simulink library "halout"  (R2021b)
settings: Solver=VariableStepAuto  StartTime=0.0  StopTime=10.0  RelTol=1e-3
undefined symbols (not defined in the file): C_TASK_5MS_S, FALSE, KHAL_CAN1FD1APS3E2E_flg, KHAL_CAN1FD1APS3TxReq_flg, KHAL_CAN1FD1VCU2E2E_flg, KHAL_CAN1FD1VCU2TxReq_flg, KHAL_CAN1FD1VCU3E2E_flg, KHAL_CAN1FD1VCU3TxReq_flg, KHAL_CAN1TxReq_flg, KHAL_CAN1VMCFCM1E2E_flg, KHAL_CAN1VMCFCM1TxReq_flg, KHAL_CAN2TxReq_flg, KHAL_CAN3FD3VCU1toNIDECTxReq_flg, KHAL_CAN3FD3VCU1TxReq_flg, KHAL_CAN3FD3VCU2E2E_flg, KHAL_CAN3FD3VCU2toNIDECE2E_flg, KHAL_CAN3FD3VCU2toNIDECTxReq_flg, KHAL_CAN3FD3VCU2TxReq_flg, KHAL_CAN3TxReq_flg, KHAL_CAN4FD4CE1000E2E_flg, KHAL_CAN4FD4CE1000TxReq_flg, KHAL_CAN4TxReq_flg, KHAL_CAN5TxReq_flg, KHAL_CAN6FD6APS3E2E_flg, KHAL_CAN6FD6APS3TxReq_flg, KHAL_CAN6FD6VCU2E2E_flg, KHAL_CAN6FD6VCU2TxReq_flg, KHAL_CAN6TxReq_flg, ONE_INT, TRUE, ZERO_INT
libraries: FVT_lib x500, simulink x235
(part 13 of 25)

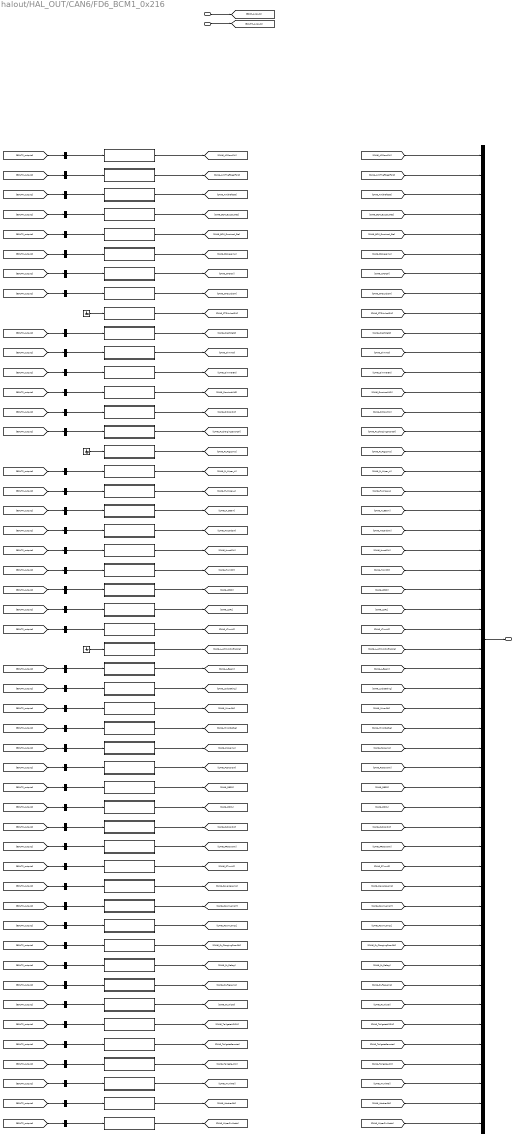
== system halout/HAL_OUT/CAN6/FD6_BCM1_0x216 ==
  BSCP_outputs : Inport  OutDataTypeStr=Bus: BSCP_outputs
  BOUTP_outputs : Inport  Port=2  OutDataTypeStr=Bus: BOUTP_outputs
  AllDoorSW : Subsystem
  AntiTheftSeatFold : Subsystem
  AntitheftSta : Subsystem
  BCMBuzzerReq : Subsystem
  BCMDoorLockSta : Subsystem
  BrakeLamp : Subsystem
  CTDCtrl : Subsystem
  CTDLockSW : Subsystem
  CTDUnlockSW : Subsystem
  CrashDetd : Subsystem
  Dimmer : Subsystem
  DimmerEN : Subsystem
  DoorLockIND : Subsystem
  DrDoorSW : Subsystem
  FrChargingDoorCtrl : Subsystem
  FrFogLamp : Subsystem
  FrWiperH : Subsystem
  FrWiperL : Subsystem
  Ground : Ground
  Ground1 : Ground
  Ground2 : Ground
  HBeam : Subsystem
  HazardSW : Subsystem
  HoodSW : Subsystem
  HornCtrl : Subsystem
  LAPMWdwEnable : Subsystem
  LBSD : Subsystem
  LBeam : Subsystem
  LDRL : Subsystem
  LTurnLP : Subsystem
  LockSetting : Subsystem
  MirrorCtrl : Subsystem
  MirrorDefog : Subsystem
  PosLamp : Subsystem
  PsDoorSW : Subsystem
  RBSD : Subsystem
  RDRL : Subsystem
  RLDoorSW : Subsystem
  RRDoorSW : Subsystem
  RTurnLP : Subsystem
  ReverseLamp : Subsystem
  RoomLampH : Subsystem
  RoomLampL : Subsystem
  RrChargingDoorCtrl : Subsystem
  RrDefog : Subsystem
  RrFogLamp : Subsystem
  RrWiper : Subsystem
  TailgateHDSW : Subsystem
  TailgateRemote : Subsystem
  TailgateSW : Subsystem
  TrunkRel : Subsystem
  WasherCtrl : Subsystem
  WiperFixMode : Subsystem
  bus_creator : BusCreator  Inputs=50  OutDataTypeStr=Bus: DT_CAN6_SG_FD6_BCM1  NonVirtualBus=on
  bus_selector : BusSelector  OutputSignals=VOUTP_AllDoorSW_flg
  bus_selector1 : BusSelector  OutputSignals=VOUTP_AntitheftSeatFlod_flg
  bus_selector10 : BusSelector  OutputSignals=VOUTP_DimmerEN_flg
  bus_selector11 : BusSelector  OutputSignals=VOUTP_DoorLockIND_flg
  bus_selector12 : BusSelector  OutputSignals=VOUTP_DrDoorSW_flg
  bus_selector13 : BusSelector  OutputSignals=VOUTP_FrChargingDoorCtrl_enum
  bus_selector14 : BusSelector  OutputSignals=VOUTP_FrWiperH_flg
  bus_selector15 : BusSelector  OutputSignals=VOUTP_FrWiperL_flg
  bus_selector16 : BusSelector  OutputSignals=VOUTP_HBeam_flg
  bus_selector17 : BusSelector  OutputSignals=VOUTP_HazardSW_flg
  bus_selector18 : BusSelector  OutputSignals=VOUTP_HoodSW_flg
  bus_selector19 : BusSelector  OutputSignals=VOUTP_HornCtrl_flg
  bus_selector2 : BusSelector  OutputSignals=VOUTP_AntitheftSta_enum
  bus_selector20 : BusSelector  OutputSignals=VOUTP_LBSD_flg
  bus_selector21 : BusSelector  OutputSignals=VOUTP_LDRL_flg
  bus_selector22 : BusSelector  OutputSignals=VOUTP_LTurnLP_flg
  bus_selector23 : BusSelector  OutputSignals=VOUTP_LBeam_flg
  bus_selector24 : BusSelector  OutputSignals=VOUTP_LockSetting_flg
  bus_selector25 : BusSelector  OutputSignals=VOUTP_MirrorCtrl_enum
  bus_selector26 : BusSelector  OutputSignals=VOUTP_MirrorDefog_flg
  bus_selector27 : BusSelector  OutputSignals=VOUTP_PosLamp_flg
  bus_selector28 : BusSelector  OutputSignals=VOUTP_PsDoorSW_flg
  bus_selector29 : BusSelector  OutputSignals=VOUTP_RBSD_flg
  bus_selector3 : BusSelector  OutputSignals=VOUTP_BCMBuzzerReq_flg
  bus_selector30 : BusSelector  OutputSignals=VOUTP_RDRL_flg
  bus_selector31 : BusSelector  OutputSignals=VOUTP_RLDoorSW_flg
  bus_selector32 : BusSelector  OutputSignals=VOUTP_RRDoorSW_flg
  bus_selector33 : BusSelector  OutputSignals=VOUTP_RTurnLP_flg
  bus_selector34 : BusSelector  OutputSignals=VOUTP_ReverseLamp_flg
  bus_selector35 : BusSelector  OutputSignals=VOUTP_RoomLampH_flg
  bus_selector36 : BusSelector  OutputSignals=VOUTP_RoomLampL_flg
  bus_selector37 : BusSelector  OutputSignals=VOUTP_RrChargingDoorCtrl_enum
  bus_selector38 : BusSelector  OutputSignals=VOUTP_RrDefog_flg
  bus_selector39 : BusSelector  OutputSignals=VOUTP_RrFogLamp_flg
  bus_selector4 : BusSelector  OutputSignals=VOUTP_BCMDoorLockSta_flg
  bus_selector40 : BusSelector  OutputSignals=VOUTP_RrWiper_flg
  bus_selector41 : BusSelector  OutputSignals=VOUTP_TailgateHDSW_flg
  bus_selector42 : BusSelector  OutputSignals=VOUTP_TailgateRemote_enum
  bus_selector43 : BusSelector  OutputSignals=VOUTP_TailgateSW_flg
  bus_selector44 : BusSelector  OutputSignals=VOUTP_TrunkRel_flg
  bus_selector45 : BusSelector  OutputSignals=VOUTP_WasherCtrl_enum
  bus_selector46 : BusSelector  OutputSignals=VOUTP_WiperFixMode_flg
  bus_selector5 : BusSelector  OutputSignals=VOUTP_BrakeLamp_flg
  bus_selector6 : BusSelector  OutputSignals=VOUTP_CTDCtrl_enum
  bus_selector7 : BusSelector  OutputSignals=VOUTP_CTDLockSW_flg
  bus_selector8 : BusSelector  OutputSignals=VOUTP_CrashDetd_flg
  bus_selector9 : BusSelector  OutputSignals=VOUTP_Dimmer_pct
  FD6_BCM1 : Outport
  wires:
  BSCP_outputs/1 -> [BSCP_outputs]
  BOUTP_outputs/1 -> [BOUTP_outputs]
  [CAN6_AllDoorSW] -> bus_creator/1  "CAN6_AllDoorSW"
  [CAN6_AntiTheftSeatFold] -> bus_creator/2  "CAN6_AntiTheftSeatFold"
  [CAN6_AntitheftSta] -> bus_creator/3  "CAN6_AntitheftSta"
  [CAN6_BCM_Buzzer_Req] -> bus_creator/4  "CAN6_BCM_Buzzer_Req"
  [CAN6_BCM_DoorLock_Sta] -> bus_creator/5  "CAN6_BCM_DoorLock_Sta"
  [CAN6_BrakeLamp] -> bus_creator/6  "CAN6_BrakeLamp"
  [CAN6_CTDCtrl] -> bus_creator/7  "CAN6_CTDCtrl"
  [CAN6_CTDLockSW] -> bus_creator/8  "CAN6_CTDLockSW"
  [CAN6_CTDUnlockSW] -> bus_creator/9  "CAN6_CTDUnlockSW"
  [CAN6_CrashDetd] -> bus_creator/10  "CAN6_CrashDetd"
  [CAN6_Dimmer] -> bus_creator/11  "CAN6_Dimmer"
  [CAN6_DimmerEN] -> bus_creator/12  "CAN6_DimmerEN"
  [CAN6_DoorLockIND] -> bus_creator/13  "CAN6_DoorLockIND"
  [CAN6_DrDoorSW] -> bus_creator/14  "CAN6_DrDoorSW"
  [CAN6_Fr_ChargingDoorCtrl] -> bus_creator/15  "CAN6_Fr_ChargingDoorCtrl"
  [CAN6_Fr_FogLamp] -> bus_creator/16  "CAN6_Fr_FogLamp"
  [CAN6_Fr_Wiper_H] -> bus_creator/17  "CAN6_Fr_Wiper_H"
  [CAN6_Fr_Wiper_L] -> bus_creator/18  "CAN6_Fr_Wiper_L"
  [CAN6_H_Beam] -> bus_creator/19  "CAN6_H_Beam"
  [CAN6_HazardSW] -> bus_creator/20  "CAN6_HazardSW"
  [CAN6_HoodSW] -> bus_creator/21  "CAN6_HoodSW"
  [CAN6_HornCtrl] -> bus_creator/22  "CAN6_HornCtrl"
  [CAN6_LBSD] -> bus_creator/23  "CAN6_LBSD"
  [CAN6_LDRL] -> bus_creator/24  "CAN6_LDRL"
  [CAN6_LTurnLP] -> bus_creator/25  "CAN6_LTurnLP"
  [CAN6_L_APM_WdwEnable] -> bus_creator/26  "CAN6_L_APM_WdwEnable"
  [CAN6_L_Beam] -> bus_creator/27  "CAN6_L_Beam"
  [CAN6_LockSetting] -> bus_creator/28  "CAN6_LockSetting"
  [CAN6_MirrorCtrl] -> bus_creator/29  "CAN6_MirrorCtrl"
  [CAN6_MirrorDefog] -> bus_creator/30  "CAN6_MirrorDefog"
  [CAN6_PosLamp] -> bus_creator/31  "CAN6_PosLamp"
  [CAN6_PsDoorSW] -> bus_creator/32  "CAN6_PsDoorSW"
  [CAN6_RBSD] -> bus_creator/33  "CAN6_RBSD"
  [CAN6_RDRL] -> bus_creator/34  "CAN6_RDRL"
  [CAN6_RLDoorSW] -> bus_creator/35  "CAN6_RLDoorSW"
  [CAN6_RRDoorSW] -> bus_creator/36  "CAN6_RRDoorSW"
  [CAN6_RTurnLP] -> bus_creator/37  "CAN6_RTurnLP"
  [CAN6_ReverseLamp] -> bus_creator/38  "CAN6_ReverseLamp"
  [CAN6_RoomLampH] -> bus_creator/39  "CAN6_RoomLampH"
  [CAN6_RoomLampL] -> bus_creator/40  "CAN6_RoomLampL"
  [CAN6_Rr_ChargingDoorCtrl] -> bus_creator/41  "CAN6_Rr_ChargingDoorCtrl"
  [CAN6_Rr_Defog] -> bus_creator/42  "CAN6_Rr_Defog"
  [CAN6_Rr_FogLamp] -> bus_creator/43  "CAN6_Rr_FogLamp"
  [CAN6_Rr_Wiper] -> bus_creator/44  "CAN6_Rr_Wiper"
  [CAN6_TailgateHDSW] -> bus_creator/45  "CAN6_TailgateHDSW"
  [CAN6_TailgateRemote] -> bus_creator/46  "CAN6_TailgateRemote"
  [CAN6_Tailgate_SW] -> bus_creator/47  "CAN6_Tailgate_SW"
  [CAN6_TrunkRel] -> bus_creator/48  "CAN6_TrunkRel"
  [CAN6_WasherCtrl] -> bus_creator/49  "CAN6_WasherCtrl"
  [CAN6_WiperFixMode] -> bus_creator/50  "CAN6_WiperFixMode"
  bus_creator/1 -> FD6_BCM1/1
  AllDoorSW/1(CAN6_AllDoorSW) -> [CAN6_AllDoorSW]
  AntiTheftSeatFold/1(CAN6_AntiTheftSeatFold) -> [CAN6_AntiTheftSeatFold]
  AntitheftSta/1(CAN6_AntitheftSta) -> [CAN6_AntitheftSta]
  BCMBuzzerReq/1(CAN6_BCM_Buzzer_Req) -> [CAN6_BCM_Buzzer_Req]
  BCMDoorLockSta/1(CAN6_BCM_DoorLock_Sta) -> [CAN6_BCM_DoorLock_Sta]
  BrakeLamp/1(CAN6_BrakeLamp) -> [CAN6_BrakeLamp]
  CTDCtrl/1(CAN6_CTDCtrl) -> [CAN6_CTDCtrl]
  CTDLockSW/1(CAN6_CTDLockSW) -> [CAN6_CTDLockSW]
  CTDUnlockSW/1(CAN6_CTDUnlockSW) -> [CAN6_CTDUnlockSW]
  CrashDetd/1(CAN6_CrashDetd) -> [CAN6_CrashDetd]
  Dimmer/1(CAN6_Dimmer) -> [CAN6_Dimmer]
  DimmerEN/1(CAN6_DimmerEN) -> [CAN6_DimmerEN]
  DoorLockIND/1(CAN6_DoorLockIND) -> [CAN6_DoorLockIND]
  DrDoorSW/1(CAN6_DrDoorSW) -> [CAN6_DrDoorSW]
  FrChargingDoorCtrl/1(CAN6_Fr_ChargingDoorCtrl) -> [CAN6_Fr_ChargingDoorCtrl]
  FrFogLamp/1(CAN6_Fr_FogLamp) -> [CAN6_Fr_FogLamp]
  FrWiperH/1(CAN6_Fr_Wiper_H) -> [CAN6_Fr_Wiper_H]
  FrWiperL/1(CAN6_Fr_Wiper_L) -> [CAN6_Fr_Wiper_L]
  HBeam/1(CAN6_H_Beam) -> [CAN6_H_Beam]
  HazardSW/1(CAN6_HazardSW) -> [CAN6_HazardSW]
  HoodSW/1(CAN6_HoodSW) -> [CAN6_HoodSW]
  HornCtrl/1(CAN6_HornCtrl) -> [CAN6_HornCtrl]
  LBSD/1(CAN6_LBSD) -> [CAN6_LBSD]
  LDRL/1(CAN6_LDRL) -> [CAN6_LDRL]
  LTurnLP/1(CAN6_LTurnLP) -> [CAN6_LTurnLP]
  LAPMWdwEnable/1(CAN6_L_APM_WdwEnable) -> [CAN6_L_APM_WdwEnable]
  LBeam/1(CAN6_L_Beam) -> [CAN6_L_Beam]
  LockSetting/1(CAN6_LockSetting) -> [CAN6_LockSetting]
  MirrorCtrl/1(CAN6_MirrorCtrl) -> [CAN6_MirrorCtrl]
  MirrorDefog/1(CAN6_MirrorDefog) -> [CAN6_MirrorDefog]
  PosLamp/1(CAN6_PosLamp) -> [CAN6_PosLamp]
  PsDoorSW/1(CAN6_PsDoorSW) -> [CAN6_PsDoorSW]
  RBSD/1(CAN6_RBSD) -> [CAN6_RBSD]
  RDRL/1(CAN6_RDRL) -> [CAN6_RDRL]
  RLDoorSW/1(CAN6_RLDoorSW) -> [CAN6_RLDoorSW]
  RRDoorSW/1(CAN6_RRDoorSW) -> [CAN6_RRDoorSW]
  RTurnLP/1(CAN6_RTurnLP) -> [CAN6_RTurnLP]
  ReverseLamp/1(CAN6_ReverseLamp) -> [CAN6_ReverseLamp]
  RoomLampH/1(CAN6_RoomLampH) -> [CAN6_RoomLampH]
  RoomLampL/1(CAN6_RoomLampL) -> [CAN6_RoomLampL]
  RrChargingDoorCtrl/1(CAN6_Rr_ChargingDoorCtrl) -> [CAN6_Rr_ChargingDoorCtrl]
  RrDefog/1(CAN6_Rr_Defog) -> [CAN6_Rr_Defog]
  RrFogLamp/1(CAN6_Rr_FogLamp) -> [CAN6_Rr_FogLamp]
  RrWiper/1(CAN6_Rr_Wiper) -> [CAN6_Rr_Wiper]
  TailgateHDSW/1(CAN6_TailgateHDSW) -> [CAN6_TailgateHDSW]
  TailgateRemote/1(CAN6_TailgateRemote) -> [CAN6_TailgateRemote]
  TailgateSW/1(CAN6_Tailgate_SW) -> [CAN6_Tailgate_SW]
  TrunkRel/1(CAN6_TrunkRel) -> [CAN6_TrunkRel]
  WasherCtrl/1(CAN6_WasherCtrl) -> [CAN6_WasherCtrl]
  WiperFixMode/1(CAN6_WiperFixMode) -> [CAN6_WiperFixMode]
  bus_selector/1 -> AllDoorSW/1(AllDoorSW)  "<VOUTP_AllDoorSW_flg>"
  [BOUTP_outputs] -> bus_selector/1
  bus_selector1/1 -> AntiTheftSeatFold/1(AntiTheftSeatFold)  "<VOUTP_AntitheftSeatFlod_flg>"
  [BOUTP_outputs] -> bus_selector1/1
  bus_selector2/1 -> AntitheftSta/1(AntitheftSta)  "<VOUTP_AntitheftSta_enum>"
  [BOUTP_outputs] -> bus_selector2/1
  bus_selector3/1 -> BCMBuzzerReq/1(BCMBuzzerReq)  "<VOUTP_BCMBuzzerReq_flg>"
  [BOUTP_outputs] -> bus_selector3/1
  bus_selector4/1 -> BCMDoorLockSta/1(BCMDoorLockSta)  "<VOUTP_BCMDoorLockSta_flg>"
  [BOUTP_outputs] -> bus_selector4/1
  bus_selector5/1 -> BrakeLamp/1(BrakeLamp)  "<VOUTP_BrakeLamp_flg>"
  [BOUTP_outputs] -> bus_selector5/1
  bus_selector6/1 -> CTDCtrl/1(CTDCtrl)  "<VOUTP_CTDCtrl_enum>"
  [BOUTP_outputs] -> bus_selector6/1
  bus_selector7/1 -> CTDLockSW/1(CTDLockSW)  "<VOUTP_CTDLockSW_flg>"
  [BOUTP_outputs] -> bus_selector7/1
  Ground/1 -> CTDUnlockSW/1(CTDUnlockSW)
  bus_selector8/1 -> CrashDetd/1(CrashDetd)  "<VOUTP_CrashDetd_flg>"
  [BOUTP_outputs] -> bus_selector8/1
  bus_selector9/1 -> Dimmer/1(Dimmer)  "<VOUTP_Dimmer_pct>"
  [BOUTP_outputs] -> bus_selector9/1
  bus_selector10/1 -> DimmerEN/1(DimmerEN)  "<VOUTP_DimmerEN_flg>"
  [BOUTP_outputs] -> bus_selector10/1
  bus_selector11/1 -> DoorLockIND/1(DoorLockIND)  "<VOUTP_DoorLockIND_flg>"
  [BOUTP_outputs] -> bus_selector11/1
  bus_selector12/1 -> DrDoorSW/1(DrDoorSW)  "<VOUTP_DrDoorSW_flg>"
  [BOUTP_outputs] -> bus_selector12/1
  bus_selector13/1 -> FrChargingDoorCtrl/1(FrChargingDoorCtrl)  "<VOUTP_FrChargingDoorCtrl_enum>"
  [BOUTP_outputs] -> bus_selector13/1
  Ground1/1 -> FrFogLamp/1(FrFogLamp)
  bus_selector14/1 -> FrWiperH/1(FrWiperH)  "<VOUTP_FrWiperH_flg>"
  [BOUTP_outputs] -> bus_selector14/1
  bus_selector15/1 -> FrWiperL/1(FrWiperL)  "<VOUTP_FrWiperL_flg>"
  [BOUTP_outputs] -> bus_selector15/1
  bus_selector16/1 -> HBeam/1(HBeam)  "<VOUTP_HBeam_flg>"
  [BOUTP_outputs] -> bus_selector16/1
  bus_selector17/1 -> HazardSW/1(HazardSW)  "<VOUTP_HazardSW_flg>"
  [BOUTP_outputs] -> bus_selector17/1
  bus_selector18/1 -> HoodSW/1(HoodSW)  "<VOUTP_HoodSW_flg>"
  [BOUTP_outputs] -> bus_selector18/1
  bus_selector19/1 -> HornCtrl/1(HornCtrl)  "<VOUTP_HornCtrl_flg>"
  [BOUTP_outputs] -> bus_selector19/1
  bus_selector20/1 -> LBSD/1(LBSD)  "<VOUTP_LBSD_flg>"
  [BOUTP_outputs] -> bus_selector20/1
  bus_selector21/1 -> LDRL/1(LDRL)  "<VOUTP_LDRL_flg>"
  [BOUTP_outputs] -> bus_selector21/1
  bus_selector22/1 -> LTurnLP/1(LTurnLP)  "<VOUTP_LTurnLP_flg>"
  [BOUTP_outputs] -> bus_selector22/1
  Ground2/1 -> LAPMWdwEnable/1(LAPMWdwEnable)
  bus_selector23/1 -> LBeam/1(LBeam)  "<VOUTP_LBeam_flg>"
  [BOUTP_outputs] -> bus_selector23/1
  bus_selector24/1 -> LockSetting/1(LockSetting)  "<VOUTP_LockSetting_flg>"
  [BOUTP_outputs] -> bus_selector24/1
  bus_selector25/1 -> MirrorCtrl/1(MirrorCtrl)  "<VOUTP_MirrorCtrl_enum>"
  [BOUTP_outputs] -> bus_selector25/1
  bus_selector26/1 -> MirrorDefog/1(MirrorDefog)  "<VOUTP_MirrorDefog_flg>"
  [BOUTP_outputs] -> bus_selector26/1
  bus_selector27/1 -> PosLamp/1(PosLamp)  "<VOUTP_PosLamp_flg>"
  [BOUTP_outputs] -> bus_selector27/1
  bus_selector28/1 -> PsDoorSW/1(PsDoorSW)  "<VOUTP_PsDoorSW_flg>"
  [BOUTP_outputs] -> bus_selector28/1
  bus_selector29/1 -> RBSD/1(RBSD)  "<VOUTP_RBSD_flg>"
  [BOUTP_outputs] -> bus_selector29/1
  bus_selector30/1 -> RDRL/1(RDRL)  "<VOUTP_RDRL_flg>"
  [BOUTP_outputs] -> bus_selector30/1
  bus_selector31/1 -> RLDoorSW/1(RLDoorSW)  "<VOUTP_RLDoorSW_flg>"
  [BOUTP_outputs] -> bus_selector31/1
  bus_selector32/1 -> RRDoorSW/1(RRDoorSW)  "<VOUTP_RRDoorSW_flg>"
  [BOUTP_outputs] -> bus_selector32/1
  bus_selector33/1 -> RTurnLP/1(RTurnLP)  "<VOUTP_RTurnLP_flg>"
  [BOUTP_outputs] -> bus_selector33/1
  bus_selector34/1 -> ReverseLamp/1(ReverseLamp)  "<VOUTP_ReverseLamp_flg>"
  [BOUTP_outputs] -> bus_selector34/1
  bus_selector35/1 -> RoomLampH/1(RoomLampH)  "<VOUTP_RoomLampH_flg>"
  [BOUTP_outputs] -> bus_selector35/1
  bus_selector36/1 -> RoomLampL/1(RoomLampL)  "<VOUTP_RoomLampL_flg>"
  [BOUTP_outputs] -> bus_selector36/1
  bus_selector37/1 -> RrChargingDoorCtrl/1(RrChargingDoorCtrl)  "<VOUTP_RrChargingDoorCtrl_enum>"
  [BOUTP_outputs] -> bus_selector37/1
  bus_selector38/1 -> RrDefog/1(RrDefog)  "<VOUTP_RrDefog_flg>"
  [BOUTP_outputs] -> bus_selector38/1
  bus_selector39/1 -> RrFogLamp/1(RrFogLamp)  "<VOUTP_RrFogLamp_flg>"
  [BOUTP_outputs] -> bus_selector39/1
  bus_selector40/1 -> RrWiper/1(RrWiper)  "<VOUTP_RrWiper_flg>"
  [BOUTP_outputs] -> bus_selector40/1
  bus_selector41/1 -> TailgateHDSW/1(TailgateHDSW)  "<VOUTP_TailgateHDSW_flg>"
  [BOUTP_outputs] -> bus_selector41/1
  bus_selector42/1 -> TailgateRemote/1(TailgateRemote)  "<VOUTP_TailgateRemote_enum>"
  [BOUTP_outputs] -> bus_selector42/1
  bus_selector43/1 -> TailgateSW/1(TailgateSW)  "<VOUTP_TailgateSW_flg>"
  [BOUTP_outputs] -> bus_selector43/1
  bus_selector44/1 -> TrunkRel/1(TrunkRel)  "<VOUTP_TrunkRel_flg>"
  [BOUTP_outputs] -> bus_selector44/1
  bus_selector45/1 -> WasherCtrl/1(WasherCtrl)  "<VOUTP_WasherCtrl_enum>"
  [BOUTP_outputs] -> bus_selector45/1
  bus_selector46/1 -> WiperFixMode/1(WiperFixMode)  "<VOUTP_WiperFixMode_flg>"
  [BOUTP_outputs] -> bus_selector46/1

== system halout/HAL_OUT/CAN6/FD6_VCU1_0x116 ==
  BSCP_outputs : Inport  OutDataTypeStr=Bus: BSCP_outputs
  BOUTP_outputs : Inport  Port=2  OutDataTypeStr=Bus: BOUTP_outputs
  CCCrlSta : Subsystem
  EngAGSCloseSta : Subsystem
  EngActvDmpDisabSta : Subsystem
  EngCoastDwSta : Subsystem
  EngPwrLockSta : Subsystem
  Ground{,1..4} (5 alike) : Ground
  HVPwrSta : Subsystem
  LVPwrSta : Subsystem
  MSACrlSta : Subsystem
  PButtonSta : Subsystem
  PrkReq : Subsystem
  PrkReqValid : Subsystem
  PwrSta : Subsystem
  ShiftGearPosn : Subsystem
  VehMalfunLevel : Subsystem
  XWDMode : Subsystem
  bus_creator : BusCreator  Inputs=15  OutDataTypeStr=Bus: DT_CAN6_SG_FD6_VCU1  NonVirtualBus=on
  bus_selector : BusSelector  OutputSignals=VOUTP_CCCtrlSta_enum
  bus_selector1 : BusSelector  OutputSignals=VOUTP_IVIPwrLockSta_enum
  bus_selector2 : BusSelector  OutputSignals=VOUTP_HVPwrSta_flg
  bus_selector3 : BusSelector  OutputSignals=VOUTP_LVPwrSta_flg
  bus_selector4 : BusSelector  OutputSignals=VOUTP_MSACtrlSta_enum
  bus_selector5 : BusSelector  OutputSignals=VOUTP_PButtonSta_enum
  bus_selector6 : BusSelector  OutputSignals=VOUTP_ActParkRequest_flg
  bus_selector7 : BusSelector  OutputSignals=VOUTP_PowerSta_enum
  bus_selector8 : BusSelector  OutputSignals=VOUTP_ShiftGearPosn_enum
  bus_selector9 : BusSelector  OutputSignals=VOUTP_DrivetrainSelect_enum
  FD6_VCU1 : Outport
  wires:
  BSCP_outputs/1 -> [BSCP_outputs]
  BOUTP_outputs/1 -> [BOUTP_outputs]
  [CAN6_CC_Crl_Sta] -> bus_creator/1  "CAN6_CC_Crl_Sta"
  [CAN6_Eng_AGSCloseSta] -> bus_creator/2  "CAN6_Eng_AGSCloseSta"
  [CAN6_Eng_ActvDmpDisabSta] -> bus_creator/3  "CAN6_Eng_ActvDmpDisabSta"
  [CAN6_Eng_CoastDwSta] -> bus_creator/4  "CAN6_Eng_CoastDwSta"
  [CAN6_Eng_PwrLockSta] -> bus_creator/5  "CAN6_Eng_PwrLockSta"
  [CAN6_HVPwrSta] -> bus_creator/6  "CAN6_HVPwrSta"
  [CAN6_LVPwrSta] -> bus_creator/7  "CAN6_LVPwrSta"
  [CAN6_MSA_Crl_Sta] -> bus_creator/8  "CAN6_MSA_Crl_Sta"
  [CAN6_P_Button_Sta] -> bus_creator/9  "CAN6_P_Button_Sta"
  [CAN6_PrkReq] -> bus_creator/10  "CAN6_PrkReq"
  [CAN6_PrkReqValid] -> bus_creator/11  "CAN6_PrkReqValid"
  [CAN6_PwrSta] -> bus_creator/12  "CAN6_PwrSta"
  [CAN6_ShiftGearPosn] -> bus_creator/13  "CAN6_ShiftGearPosn"
  [CAN6_VehMalfunLevel] -> bus_creator/14  "CAN6_VehMalfunLevel"
  [CAN6_XWDMode] -> bus_creator/15  "CAN6_XWDMode"
  bus_creator/1 -> FD6_VCU1/1
  CCCrlSta/1(CAN6_CC_Crl_Sta) -> [CAN6_CC_Crl_Sta]
  EngAGSCloseSta/1(CAN6_Eng_AGSCloseSta) -> [CAN6_Eng_AGSCloseSta]
  EngActvDmpDisabSta/1(CAN6_Eng_ActvDmpDisabSta) -> [CAN6_Eng_ActvDmpDisabSta]
  EngCoastDwSta/1(CAN6_Eng_CoastDwSta) -> [CAN6_Eng_CoastDwSta]
  EngPwrLockSta/1(CAN6_Eng_PwrLockSta) -> [CAN6_Eng_PwrLockSta]
  HVPwrSta/1(CAN6_HVPwrSta) -> [CAN6_HVPwrSta]
  LVPwrSta/1(CAN6_LVPwrSta) -> [CAN6_LVPwrSta]
  MSACrlSta/1(CAN6_MSA_Crl_Sta) -> [CAN6_MSA_Crl_Sta]
  PButtonSta/1(CAN6_P_Button_Sta) -> [CAN6_P_Button_Sta]
  PrkReq/1(CAN6_PrkReq) -> [CAN6_PrkReq]
  PrkReqValid/1(CAN6_PrkReqValid) -> [CAN6_PrkReqValid]
  PwrSta/1(CAN6_PwrSta) -> [CAN6_PwrSta]
  ShiftGearPosn/1(CAN6_ShiftGearPosn) -> [CAN6_ShiftGearPosn]
  VehMalfunLevel/1(CAN6_VehMalfunLevel) -> [CAN6_VehMalfunLevel]
  XWDMode/1(CAN6_XWDMode) -> [CAN6_XWDMode]
  bus_selector/1 -> CCCrlSta/1(CCCrlSta)  "<VOUTP_CCCtrlSta_enum>"
  [BOUTP_outputs] -> bus_selector/1
  Ground/1 -> EngAGSCloseSta/1(EngAGSCloseSta)
  Ground1/1 -> EngActvDmpDisabSta/1(EngActvDmpDisabSta)
  Ground2/1 -> EngCoastDwSta/1(EngCoastDwSta)
  bus_selector1/1 -> EngPwrLockSta/1(EngPwrLockSta)  "<VOUTP_IVIPwrLockSta_enum>"
  [BOUTP_outputs] -> bus_selector1/1
  bus_selector2/1 -> HVPwrSta/1(HVPwrSta)  "<VOUTP_HVPwrSta_flg>"
  [BOUTP_outputs] -> bus_selector2/1
  bus_selector3/1 -> LVPwrSta/1(LVPwrSta)  "<VOUTP_LVPwrSta_flg>"
  [BOUTP_outputs] -> bus_selector3/1
  bus_selector4/1 -> MSACrlSta/1(MSACrlSta)  "<VOUTP_MSACtrlSta_enum>"
  [BOUTP_outputs] -> bus_selector4/1
  bus_selector5/1 -> PButtonSta/1(PButtonSta)  "<VOUTP_PButtonSta_enum>"
  [BOUTP_outputs] -> bus_selector5/1
  bus_selector6/1 -> PrkReq/1(PrkReq)  "<VOUTP_ActParkRequest_flg>"
  [BOUTP_outputs] -> bus_selector6/1
  Ground3/1 -> PrkReqValid/1(PrkReqValid)
  bus_selector7/1 -> PwrSta/1(PwrSta)  "<VOUTP_PowerSta_enum>"
  [BOUTP_outputs] -> bus_selector7/1
  bus_selector8/1 -> ShiftGearPosn/1(ShiftGearPosn)  "<VOUTP_ShiftGearPosn_enum>"
  [BOUTP_outputs] -> bus_selector8/1
  Ground4/1 -> VehMalfunLevel/1(VehMalfunLevel)
  bus_selector9/1 -> XWDMode/1(XWDMode)  "<VOUTP_DrivetrainSelect_enum>"
  [BOUTP_outputs] -> bus_selector9/1

== system halout/HAL_OUT/CAN6/FD6_VCU2_0x154 ==
  BSCP_outputs : Inport  OutDataTypeStr=Bus: BSCP_outputs
  BOUTP_outputs : Inport  Port=2  OutDataTypeStr=Bus: BOUTP_outputs
  Trigger : TriggerPort  TriggerType=function-call  VariantControl=(inherit)
  ACCCtrlAvail : Subsystem
  AccPedalOverride : Subsystem
  ActAPSPosn : Subsystem
  Byte_0 : Subsystem
  Byte_1 : Subsystem
  Byte_10 : Subsystem
  Byte_11 : Subsystem
  Byte_12 : Subsystem
  Byte_13 : Subsystem
  Byte_14 : Subsystem
  Byte_15 : Subsystem
  Byte_2 : Subsystem
  Byte_3 : Subsystem
  Byte_4 : Subsystem
  Byte_5 : Subsystem
  Byte_6 : Subsystem
  Byte_7 : Constant  Value=ZERO_INT
  Byte_8 : Constant  Value=ZERO_INT
  Byte_9 : Constant  Value=ZERO_INT
  CRC8_IfAction_Tx : Subsystem  AncestorBlock=FVT_lib/hal/CRC8_IfAction_Tx
      mask help: MeasumentTrigerEvent
      mask Display: fprintf('CRC8_IfAction');
  CSVCU2CAN6 : Subsystem
  Constant : Constant  Value=KHAL_CAN6FD6VCU2E2E_flg
  Constant1 : Constant  Value=0x32
  Constant2 : Constant  Value=0xBF
  Constant3 : Constant  Value=KHAL_CAN6FD6VCU2E2E_flg
  Constant4 : Constant  Value=KHAL_CAN6FD6VCU2E2E_flg
  DriverTq : Subsystem
  FrDriverTq : Subsystem
  Ground{,1..7} (8 alike) : Ground
  Mux2 : Mux  Inputs=15
  RCVCU2CAN6 : Subsystem
  RollingCounter_IfAction : FVT_lib/hal/RollingCounter_IfAction
  RollingCounter_IfAction1 : FVT_lib/hal/RollingCounter_IfAction
  RrDriverTq : Subsystem
  Terminator : Terminator
  VehActPwr : Subsystem
  bus_creator : BusCreator  Inputs=9  OutDataTypeStr=Bus: DT_CAN6_SG_FD6_VCU2  NonVirtualBus=on
  bus_selector : BusSelector  OutputSignals=VOUTP_DriverWhlTqDemFr_Nm
  bus_selector1 : BusSelector  OutputSignals=VOUTP_DriverWhlTqDemFr_Nm
  bus_selector10 : BusSelector  OutputSignals=VOUTP_DriverWhlTqDemFr_Nm
  bus_selector11 : BusSelector  OutputSignals=VOUTP_DriverWhlTqDemRr_Nm
  bus_selector2 : BusSelector  OutputSignals=VOUTP_DriverWhlTqDemRr_Nm
  bus_selector3 : BusSelector  OutputSignals=VOUTP_DriverWhlTqDemRr_Nm
  bus_selector4 : BusSelector  OutputSignals=VOUTP_ACCCtrlAvail_flg
  bus_selector5 : BusSelector  OutputSignals=VOUTP_ACCPedalOvrd_flg
  bus_selector6 : BusSelector  OutputSignals=VOUTP_ActAPSPosn_pct
  bus_selector7 : BusSelector  OutputSignals=VOUTP_ACCCtrlAvail_flg
  bus_selector8 : BusSelector  OutputSignals=VOUTP_ACCPedalOvrd_flg
  bus_selector9 : BusSelector  OutputSignals=VOUTP_ActAPSPosn_pct
  FD6_VCU2 : Outport
  wires:
  BSCP_outputs/1 -> [BSCP_outputs]
  BOUTP_outputs/1 -> [BOUTP_outputs]
  [CAN6_ACC_CtrlAvail] -> bus_creator/1  "CAN6_ACC_CtrlAvail"
  [CAN6_AccPedal_Override] -> bus_creator/2  "CAN6_AccPedal_Override"
  [CAN6_ActAPSPosn] -> bus_creator/3  "CAN6_ActAPSPosn"
  [CAN6_CS_VCU2_CAN6] -> bus_creator/4  "CAN6_CS_VCU2_CAN6"
  [CAN6_DriverTq] -> bus_creator/5  "CAN6_DriverTq"
  [CAN6_Fr_DriverTq] -> bus_creator/6  "CAN6_Fr_DriverTq"
  [CAN6_RC_VCU2_CAN6] -> bus_creator/7  "CAN6_RC_VCU2_CAN6"
  [CAN6_Rr_DriverTq] -> bus_creator/8  "CAN6_Rr_DriverTq"
  [CAN6_VehActPwr] -> bus_creator/9  "CAN6_VehActPwr"
  bus_creator/1 -> FD6_VCU2/1
  ACCCtrlAvail/1(CAN6_ACC_CtrlAvail) -> [CAN6_ACC_CtrlAvail]
  AccPedalOverride/1(CAN6_AccPedal_Override) -> [CAN6_AccPedal_Override]
  ActAPSPosn/1(CAN6_ActAPSPosn) -> [CAN6_ActAPSPosn]
  CSVCU2CAN6/1(CAN6_CS_VCU2_CAN6) -> [CAN6_CS_VCU2_CAN6]
  DriverTq/1(CAN6_DriverTq) -> [CAN6_DriverTq]
  FrDriverTq/1(CAN6_Fr_DriverTq) -> [CAN6_Fr_DriverTq]
  RCVCU2CAN6/1(CAN6_RC_VCU2_CAN6) -> [CAN6_RC_VCU2_CAN6]
  RrDriverTq/1(CAN6_Rr_DriverTq) -> [CAN6_Rr_DriverTq]
  VehActPwr/1(CAN6_VehActPwr) -> [CAN6_VehActPwr]
  Byte_0/1(Byte_0) -> Terminator/1
  Byte_1/1(Byte_1) -> [Byte_1]
  Byte_2/1(Byte_2) -> [Byte_2]
  Byte_3/1(Byte_3) -> [Byte_3]
  Byte_4/1(Byte_4) -> [Byte_4]
  Byte_5/1(Byte_5) -> [Byte_5]
  Byte_6/1(Byte_6) -> [Byte_6]
  Byte_7/1 -> [Byte_7]
  Byte_8/1 -> [Byte_8]
  Byte_9/1 -> [Byte_9]
  Byte_10/1(Byte_10) -> [Byte_10]
  Byte_11/1(Byte_11) -> [Byte_11]
  Byte_12/1(Byte_12) -> [Byte_12]
  Byte_13/1(Byte_13) -> [Byte_13]
  Byte_14/1(Byte_14) -> [Byte_14]
  Byte_15/1(Byte_15) -> [Byte_15]
  Mux2/1 -> CRC8_IfAction_Tx/4(RawData)
  Constant/1 -> CRC8_IfAction_Tx/1(CAN_E2E_flg)
  Constant1/1 -> CRC8_IfAction_Tx/2(DataID1)
  Constant2/1 -> CRC8_IfAction_Tx/3(DataID2)
  CRC8_IfAction_Tx/1(CRC8) -> [CS_VCU2_CAN6]
  Ground/1 -> Byte_0/1(CS_VCU2_CAN6)
  [Byte_1] -> Mux2/1
  RollingCounter_IfAction/1 -> Byte_1/1(RC_VCU2_CAN6)
  Constant3/1 -> RollingCounter_IfAction/1
  [Byte_2] -> Mux2/2
  bus_selector/1 -> Byte_2/1(Fr_DriverTq)  "<VOUTP_DriverWhlTqDemFr_Nm>"
  [BOUTP_outputs] -> bus_selector/1
  [Byte_3] -> Mux2/3
  bus_selector1/1 -> Byte_3/1(Fr_DriverTq)  "<VOUTP_DriverWhlTqDemFr_Nm>"
  [BOUTP_outputs] -> bus_selector1/1
  [Byte_4] -> Mux2/4
  bus_selector2/1 -> Byte_4/1(Rr_DriverTq)  "<VOUTP_DriverWhlTqDemRr_Nm>"
  [BOUTP_outputs] -> bus_selector2/1
  [Byte_5] -> Mux2/5
  bus_selector3/1 -> Byte_5/1(Rr_DriverTq)  "<VOUTP_DriverWhlTqDemRr_Nm>"
  [BOUTP_outputs] -> bus_selector3/1
  [Byte_6] -> Mux2/6
  bus_selector4/1 -> Byte_6/1(ACC_CtrlAvail)  "<VOUTP_ACCCtrlAvail_flg>"
  [BOUTP_outputs] -> bus_selector4/1
  bus_selector5/1 -> Byte_6/2(AccPedal_Override)  "<VOUTP_ACCPedalOvrd_flg>"
  [BOUTP_outputs] -> bus_selector5/1
  [Byte_7] -> Mux2/7
  [Byte_8] -> Mux2/8
  [Byte_9] -> Mux2/9
  [Byte_10] -> Mux2/10
  Ground1/1 -> Byte_10/1(VehActPwr)
  [Byte_11] -> Mux2/11
  Ground2/1 -> Byte_11/1(VehActPwr)
  [Byte_12] -> Mux2/12
  Ground3/1 -> Byte_12/1(VehActPwr)
  [Byte_13] -> Mux2/13
  Ground4/1 -> Byte_13/1(DriverTq)
  [Byte_14] -> Mux2/14
  Ground5/1 -> Byte_14/1(DriverTq)
  [Byte_15] -> Mux2/15
  bus_selector6/1 -> Byte_15/1(ActAPSPosn)  "<VOUTP_ActAPSPosn_pct>"
  [BOUTP_outputs] -> bus_selector6/1
  bus_selector7/1 -> ACCCtrlAvail/1(ACCCtrlAvail)  "<VOUTP_ACCCtrlAvail_flg>"
  [BOUTP_outputs] -> bus_selector7/1
  bus_selector8/1 -> AccPedalOverride/1(AccPedalOverride)  "<VOUTP_ACCPedalOvrd_flg>"
  [BOUTP_outputs] -> bus_selector8/1
  bus_selector9/1 -> ActAPSPosn/1(ActAPSPosn)  "<VOUTP_ActAPSPosn_pct>"
  [BOUTP_outputs] -> bus_selector9/1
  [CS_VCU2_CAN6] -> CSVCU2CAN6/1(CSVCU2CAN6)
  Ground6/1 -> DriverTq/1(DriverTq)
  bus_selector10/1 -> FrDriverTq/1(FrDriverTq)  "<VOUTP_DriverWhlTqDemFr_Nm>"
  [BOUTP_outputs] -> bus_selector10/1
  RollingCounter_IfAction1/1 -> RCVCU2CAN6/1(RCVCU2CAN6)
  Constant4/1 -> RollingCounter_IfAction1/1
  bus_selector11/1 -> RrDriverTq/1(RrDriverTq)  "<VOUTP_DriverWhlTqDemRr_Nm>"
  [BOUTP_outputs] -> bus_selector11/1
  Ground7/1 -> VehActPwr/1(VehActPwr)

== system halout/HAL_OUT/CAN6/FD6_VCU2_Tx ==
  TxReq : Inport
  Chart : Stateflow chart  TreatAsAtomicUnit=on
  Constant : Constant  Value=C_TASK_5MS_S
  Constant3 : Constant  Value=CycleTime
  Data Type Conversion : DataTypeConversion  OutDataTypeStr=uint16
  Divide : Product  Inputs=*/
  Gain : Gain  Gain=0.001
  TxTrigger : Outport
  wires:
  Data Type Conversion/1 -> Chart/2(CycleCnt)
  Constant3/1 -> Gain/1
  Gain/1 -> Divide/1
  Chart/1(TxTrigger()) -> TxTrigger/1
  Divide/1 -> Data Type Conversion/1
  TxReq/1 -> Chart/1(TxReq)
  Constant/1 -> Divide/2

== system halout/HAL_OUT/CAN6/FD6_VMC1_0x17F ==
  BSCP_outputs : Inport  OutDataTypeStr=Bus: BSCP_outputs
  BOUTP_outputs : Inport  Port=2  OutDataTypeStr=Bus: BOUTP_outputs
  AccCalcuPID : Subsystem
  CCMSASpdWar : Subsystem
  DISCButtSta : Subsystem
  DISCDISCTargetSpd : Subsystem
  DISCDISCTurn : Subsystem
  DISCReqAcc : Subsystem
  DISCSta : Subsystem
  FeatArbitrFinal : Subsystem
  FeatArbitrSta : Subsystem
  FeatReqSpd : Subsystem
  FeatSetSpdFinalraw32 : Subsystem
  FrontRearSlipRatioCtrl : Subsystem
  Ground : Ground
  Ground1 : Ground
  ISOAccLimit : Subsystem
  ISODecLimit : Subsystem
  ISOJerkLimit : Subsystem
  JerkPCT : Subsystem
  LatAccCtrl : Subsystem
  LateralCtrl : Subsystem
  LimitPCT : Subsystem
  MeterIndSpeedraw32 : Subsystem
  RearWhlSlipRatioCtrl : Subsystem
  SPD2ACCAct : Subsystem
  SafetyCtrl : Subsystem
  SingleWhlSlipRatioCtrl : Subsystem
  TimeGapCalcu : Subsystem
  VMCACCCtrlAvail : Subsystem
  VMCAEBCtrlAvail : Subsystem
  VMCCCCtrlAvail : Subsystem
  VMCMSACtrlAvail : Subsystem
  VMCVCUACCCtrlAvail : Subsystem
  VMCVCUAPSCtrlAvailflg : Subsystem
  VMCVCUAccPedalOverride : Subsystem
  VMCVCUCCCrlSta : Subsystem
  VMCVCUMSACrlSta : Subsystem
  VehicleSpeedkph : Subsystem
  VehicleSpeedmph : Subsystem
  bus_creator : BusCreator  Inputs=36  OutDataTypeStr=Bus: DT_CAN6_SG_FD6_VMC1  NonVirtualBus=on
  bus_selector : BusSelector  OutputSignals=VOUTP_AccCalcuPID_mps2
  bus_selector1 : BusSelector  OutputSignals=VOUTP_CCMSASpdWar_flg
  bus_selector10 : BusSelector  OutputSignals=VOUTP_FeatSetSpdFinal_raw32
  bus_selector11 : BusSelector  OutputSignals=VOUTP_FrontRearSlipRatioCtrl_flg
  bus_selector12 : BusSelector  OutputSignals=VOUTP_ISOAccLimit_mps2
  bus_selector13 : BusSelector  OutputSignals=VOUTP_ISODecLimit_mps2
  bus_selector14 : BusSelector  OutputSignals=VOUTP_ISOJerkLimit_mps3
  bus_selector15 : BusSelector  OutputSignals=VOUTP_JerkPCT_pct
  bus_selector16 : BusSelector  OutputSignals=VOUTP_LatAccCtrl_flg
  bus_selector17 : BusSelector  OutputSignals=VOUTP_LateralCtrl_flg
  bus_selector18 : BusSelector  OutputSignals=VOUTP_LimitPCT_pct
  bus_selector19 : BusSelector  OutputSignals=VOUTP_MeterIndSpeed_raw32
  bus_selector2 : BusSelector  OutputSignals=VOUTP_DISCReqAcc_mps2
  bus_selector20 : BusSelector  OutputSignals=VOUTP_RearWhlSlipRatioCtrl_flg
  bus_selector21 : BusSelector  OutputSignals=VOUTP_SPD2ACCAct_flg
  bus_selector22 : BusSelector  OutputSignals=VOUTP_SafetyCtrl_flg
  bus_selector23 : BusSelector  OutputSignals=VOUTP_SingleWhlSlipRatioCtrl_flg
  bus_selector24 : BusSelector  OutputSignals=VOUTP_TimeGapCalcu_s
  bus_selector25 : BusSelector  OutputSignals=VOUTP_VMCACCCtrlAvail_flg
  bus_selector26 : BusSelector  OutputSignals=VOUTP_VMCAEBCtrlAvail_flg
  bus_selector27 : BusSelector  OutputSignals=VOUTP_VMCCCCtrlAvail_flg
  bus_selector28 : BusSelector  OutputSignals=VOUTP_VMCMSACtrlAvail_flg
  bus_selector29 : BusSelector  OutputSignals=VOUTP_ACCCtrlAvail_flg
  bus_selector3 : BusSelector  OutputSignals=VOUTP_DISCButtSta_flg
  bus_selector30 : BusSelector  OutputSignals=VOUTP_APSCtrlAvail_flg
  bus_selector31 : BusSelector  OutputSignals=VOUTP_ACCPedalOvrd_flg
  bus_selector32 : BusSelector  OutputSignals=VOUTP_CCCtrlSta_enum
  bus_selector33 : BusSelector  OutputSignals=VOUTP_MSACtrlSta_enum
  bus_selector4 : BusSelector  OutputSignals=VOUTP_DISCTargetSpd_kph
  bus_selector5 : BusSelector  OutputSignals=VOUTP_DISCTurn_flg
  bus_selector6 : BusSelector  OutputSignals=VOUTP_DISCSta_enum
  bus_selector7 : BusSelector  OutputSignals=VOUTP_FeatArbitrFinal_enum
  bus_selector8 : BusSelector  OutputSignals=VOUTP_FeatArbitrSta_enum
  bus_selector9 : BusSelector  OutputSignals=VOUTP_FeatReqSpd_kph
  FD6_VMC1 : Outport
  wires:
  BSCP_outputs/1 -> [BSCP_outputs]
  BOUTP_outputs/1 -> [BOUTP_outputs]
  [CAN6_AccCalcuPID] -> bus_creator/1  "CAN6_AccCalcuPID"
  [CAN6_CCMSA_SpdWar] -> bus_creator/2  "CAN6_CCMSA_SpdWar"
  [CAN6_DISCReqAcc] -> bus_creator/3  "CAN6_DISCReqAcc"
  [CAN6_DISC_ButtSta] -> bus_creator/4  "CAN6_DISC_ButtSta"
  [CAN6_DISC_DISCTargetSpd] -> bus_creator/5  "CAN6_DISC_DISCTargetSpd"
  [CAN6_DISC_DISCTurn] -> bus_creator/6  "CAN6_DISC_DISCTurn"
  [CAN6_DISC_Sta] -> bus_creator/7  "CAN6_DISC_Sta"
  [CAN6_FeatArbitrFinal] -> bus_creator/8  "CAN6_FeatArbitrFinal"
  [CAN6_FeatArbitrSta] -> bus_creator/9  "CAN6_FeatArbitrSta"
  [CAN6_FeatReqSpd] -> bus_creator/10  "CAN6_FeatReqSpd"
  [CAN6_FeatSetSpdFinal_raw32] -> bus_creator/11  "CAN6_FeatSetSpdFinal_raw32"
  [CAN6_FrontRearSlipRatioCtrl] -> bus_creator/12  "CAN6_FrontRearSlipRatioCtrl"
  [CAN6_ISOAccLimit] -> bus_creator/13  "CAN6_ISOAccLimit"
  [CAN6_ISODecLimit] -> bus_creator/14  "CAN6_ISODecLimit"
  [CAN6_ISOJerkLimit] -> bus_creator/15  "CAN6_ISOJerkLimit"
  [CAN6_JerkPCT] -> bus_creator/16  "CAN6_JerkPCT"
  [CAN6_LatAccCtrl] -> bus_creator/17  "CAN6_LatAccCtrl"
  [CAN6_LateralCtrl] -> bus_creator/18  "CAN6_LateralCtrl"
  [CAN6_LimitPCT] -> bus_creator/19  "CAN6_LimitPCT"
  [CAN6_MeterIndSpeed_raw32] -> bus_creator/20  "CAN6_MeterIndSpeed_raw32"
  [CAN6_RearWhlSlipRatioCtrl] -> bus_creator/21  "CAN6_RearWhlSlipRatioCtrl"
  [CAN6_SPD2ACCAct] -> bus_creator/22  "CAN6_SPD2ACCAct"
  [CAN6_SafetyCtrl] -> bus_creator/23  "CAN6_SafetyCtrl"
  [CAN6_SingleWhlSlipRatioCtrl] -> bus_creator/24  "CAN6_SingleWhlSlipRatioCtrl"
  [CAN6_TimeGapCalcu] -> bus_creator/25  "CAN6_TimeGapCalcu"
  [CAN6_VMC_ACCCtrlAvail] -> bus_creator/26  "CAN6_VMC_ACCCtrlAvail"
  [CAN6_VMC_AEBCtrlAvail] -> bus_creator/27  "CAN6_VMC_AEBCtrlAvail"
  [CAN6_VMC_CCCtrlAvail] -> bus_creator/28  "CAN6_VMC_CCCtrlAvail"
  [CAN6_VMC_MSACtrlAvail] -> bus_creator/29  "CAN6_VMC_MSACtrlAvail"
  [CAN6_VMC_VCU_ACC_CtrlAvail] -> bus_creator/30  "CAN6_VMC_VCU_ACC_CtrlAvail"
  [CAN6_VMC_VCU_APSCtrlAvail_flg] -> bus_creator/31  "CAN6_VMC_VCU_APSCtrlAvail_flg"
  [CAN6_VMC_VCU_AccPedal_Override] -> bus_creator/32  "CAN6_VMC_VCU_AccPedal_Override"
  [CAN6_VMC_VCU_CC_Crl_Sta] -> bus_creator/33  "CAN6_VMC_VCU_CC_Crl_Sta"
  [CAN6_VMC_VCU_MSA_Crl_Sta] -> bus_creator/34  "CAN6_VMC_VCU_MSA_Crl_Sta"
  [CAN6_VehicleSpeed_kph] -> bus_creator/35  "CAN6_VehicleSpeed_kph"
  [CAN6_VehicleSpeed_mph] -> bus_creator/36  "CAN6_VehicleSpeed_mph"
  bus_creator/1 -> FD6_VMC1/1
  AccCalcuPID/1(CAN6_AccCalcuPID) -> [CAN6_AccCalcuPID]
  CCMSASpdWar/1(CAN6_CCMSA_SpdWar) -> [CAN6_CCMSA_SpdWar]
  DISCReqAcc/1(CAN6_DISCReqAcc) -> [CAN6_DISCReqAcc]
  DISCButtSta/1(CAN6_DISC_ButtSta) -> [CAN6_DISC_ButtSta]
  DISCDISCTargetSpd/1(CAN6_DISC_DISCTargetSpd) -> [CAN6_DISC_DISCTargetSpd]
  DISCDISCTurn/1(CAN6_DISC_DISCTurn) -> [CAN6_DISC_DISCTurn]
  DISCSta/1(CAN6_DISC_Sta) -> [CAN6_DISC_Sta]
  FeatArbitrFinal/1(CAN6_FeatArbitrFinal) -> [CAN6_FeatArbitrFinal]
  FeatArbitrSta/1(CAN6_FeatArbitrSta) -> [CAN6_FeatArbitrSta]
  FeatReqSpd/1(CAN6_FeatReqSpd) -> [CAN6_FeatReqSpd]
  FeatSetSpdFinalraw32/1(CAN6_FeatSetSpdFinal_raw32) -> [CAN6_FeatSetSpdFinal_raw32]
  FrontRearSlipRatioCtrl/1(CAN6_FrontRearSlipRatioCtrl) -> [CAN6_FrontRearSlipRatioCtrl]
  ISOAccLimit/1(CAN6_ISOAccLimit) -> [CAN6_ISOAccLimit]
  ISODecLimit/1(CAN6_ISODecLimit) -> [CAN6_ISODecLimit]
  ISOJerkLimit/1(CAN6_ISOJerkLimit) -> [CAN6_ISOJerkLimit]
  JerkPCT/1(CAN6_JerkPCT) -> [CAN6_JerkPCT]
  LatAccCtrl/1(CAN6_LatAccCtrl) -> [CAN6_LatAccCtrl]
  LateralCtrl/1(CAN6_LateralCtrl) -> [CAN6_LateralCtrl]
  LimitPCT/1(CAN6_LimitPCT) -> [CAN6_LimitPCT]
  MeterIndSpeedraw32/1(CAN6_MeterIndSpeed_raw32) -> [CAN6_MeterIndSpeed_raw32]
  RearWhlSlipRatioCtrl/1(CAN6_RearWhlSlipRatioCtrl) -> [CAN6_RearWhlSlipRatioCtrl]
  SPD2ACCAct/1(CAN6_SPD2ACCAct) -> [CAN6_SPD2ACCAct]
  SafetyCtrl/1(CAN6_SafetyCtrl) -> [CAN6_SafetyCtrl]
  SingleWhlSlipRatioCtrl/1(CAN6_SingleWhlSlipRatioCtrl) -> [CAN6_SingleWhlSlipRatioCtrl]
  TimeGapCalcu/1(CAN6_TimeGapCalcu) -> [CAN6_TimeGapCalcu]
  VMCACCCtrlAvail/1(CAN6_VMC_ACCCtrlAvail) -> [CAN6_VMC_ACCCtrlAvail]
  VMCAEBCtrlAvail/1(CAN6_VMC_AEBCtrlAvail) -> [CAN6_VMC_AEBCtrlAvail]
  VMCCCCtrlAvail/1(CAN6_VMC_CCCtrlAvail) -> [CAN6_VMC_CCCtrlAvail]
  VMCMSACtrlAvail/1(CAN6_VMC_MSACtrlAvail) -> [CAN6_VMC_MSACtrlAvail]
  VMCVCUACCCtrlAvail/1(CAN6_VMC_VCU_ACC_CtrlAvail) -> [CAN6_VMC_VCU_ACC_CtrlAvail]
  VMCVCUAPSCtrlAvailflg/1(CAN6_VMC_VCU_APSCtrlAvail_flg) -> [CAN6_VMC_VCU_APSCtrlAvail_flg]
  VMCVCUAccPedalOverride/1(CAN6_VMC_VCU_AccPedal_Override) -> [CAN6_VMC_VCU_AccPedal_Override]
  VMCVCUCCCrlSta/1(CAN6_VMC_VCU_CC_Crl_Sta) -> [CAN6_VMC_VCU_CC_Crl_Sta]
  VMCVCUMSACrlSta/1(CAN6_VMC_VCU_MSA_Crl_Sta) -> [CAN6_VMC_VCU_MSA_Crl_Sta]
  VehicleSpeedkph/1(CAN6_VehicleSpeed_kph) -> [CAN6_VehicleSpeed_kph]
  VehicleSpeedmph/1(CAN6_VehicleSpeed_mph) -> [CAN6_VehicleSpeed_mph]
  bus_selector/1 -> AccCalcuPID/1(AccCalcuPID)  "<VOUTP_AccCalcuPID_mps2>"
  [BOUTP_outputs] -> bus_selector/1
  bus_selector1/1 -> CCMSASpdWar/1(CCMSASpdWar)  "<VOUTP_CCMSASpdWar_flg>"
  [BOUTP_outputs] -> bus_selector1/1
  bus_selector2/1 -> DISCReqAcc/1(DISCReqAcc)  "<VOUTP_DISCReqAcc_mps2>"
  [BOUTP_outputs] -> bus_selector2/1
  bus_selector3/1 -> DISCButtSta/1(DISCButtSta)  "<VOUTP_DISCButtSta_flg>"
  [BOUTP_outputs] -> bus_selector3/1
  bus_selector4/1 -> DISCDISCTargetSpd/1(DISCDISCTargetSpd)  "<VOUTP_DISCTargetSpd_kph>"
  [BOUTP_outputs] -> bus_selector4/1
  bus_selector5/1 -> DISCDISCTurn/1(DISCDISCTurn)  "<VOUTP_DISCTurn_flg>"
  [BOUTP_outputs] -> bus_selector5/1
  bus_selector6/1 -> DISCSta/1(DISCSta)  "<VOUTP_DISCSta_enum>"
  [BOUTP_outputs] -> bus_selector6/1
  bus_selector7/1 -> FeatArbitrFinal/1(FeatArbitrFinal)  "<VOUTP_FeatArbitrFinal_enum>"
  [BOUTP_outputs] -> bus_selector7/1
  bus_selector8/1 -> FeatArbitrSta/1(FeatArbitrSta)  "<VOUTP_FeatArbitrSta_enum>"
  [BOUTP_outputs] -> bus_selector8/1
  bus_selector9/1 -> FeatReqSpd/1(FeatReqSpd)  "<VOUTP_FeatReqSpd_kph>"
  [BOUTP_outputs] -> bus_selector9/1
  bus_selector10/1 -> FeatSetSpdFinalraw32/1(FeatSetSpdFinalraw32)  "<VOUTP_FeatSetSpdFinal_raw32>"
  [BOUTP_outputs] -> bus_selector10/1
  bus_selector11/1 -> FrontRearSlipRatioCtrl/1(FrontRearSlipRatioCtrl)  "<VOUTP_FrontRearSlipRatioCtrl_flg>"
  [BOUTP_outputs] -> bus_selector11/1
  bus_selector12/1 -> ISOAccLimit/1(ISOAccLimit)  "<VOUTP_ISOAccLimit_mps2>"
  [BOUTP_outputs] -> bus_selector12/1
  bus_selector13/1 -> ISODecLimit/1(ISODecLimit)  "<VOUTP_ISODecLimit_mps2>"
  [BOUTP_outputs] -> bus_selector13/1
  bus_selector14/1 -> ISOJerkLimit/1(ISOJerkLimit)  "<VOUTP_ISOJerkLimit_mps3>"
  [BOUTP_outputs] -> bus_selector14/1
  bus_selector15/1 -> JerkPCT/1(JerkPCT)  "<VOUTP_JerkPCT_pct>"
  [BOUTP_outputs] -> bus_selector15/1
  bus_selector16/1 -> LatAccCtrl/1(LatAccCtrl)  "<VOUTP_LatAccCtrl_flg>"
  [BOUTP_outputs] -> bus_selector16/1
  bus_selector17/1 -> LateralCtrl/1(LateralCtrl)  "<VOUTP_LateralCtrl_flg>"
  [BOUTP_outputs] -> bus_selector17/1
  bus_selector18/1 -> LimitPCT/1(LimitPCT)  "<VOUTP_LimitPCT_pct>"
  [BOUTP_outputs] -> bus_selector18/1
  bus_selector19/1 -> MeterIndSpeedraw32/1(MeterIndSpeedraw32)  "<VOUTP_MeterIndSpeed_raw32>"
  [BOUTP_outputs] -> bus_selector19/1
  bus_selector20/1 -> RearWhlSlipRatioCtrl/1(RearWhlSlipRatioCtrl)  "<VOUTP_RearWhlSlipRatioCtrl_flg>"
  [BOUTP_outputs] -> bus_selector20/1
  bus_selector21/1 -> SPD2ACCAct/1(SPD2ACCAct)  "<VOUTP_SPD2ACCAct_flg>"
  [BOUTP_outputs] -> bus_selector21/1
  bus_selector22/1 -> SafetyCtrl/1(SafetyCtrl)  "<VOUTP_SafetyCtrl_flg>"
  [BOUTP_outputs] -> bus_selector22/1
  bus_selector23/1 -> SingleWhlSlipRatioCtrl/1(SingleWhlSlipRatioCtrl)  "<VOUTP_SingleWhlSlipRatioCtrl_flg>"
  [BOUTP_outputs] -> bus_selector23/1
  bus_selector24/1 -> TimeGapCalcu/1(TimeGapCalcu)  "<VOUTP_TimeGapCalcu_s>"
  [BOUTP_outputs] -> bus_selector24/1
  bus_selector25/1 -> VMCACCCtrlAvail/1(VMCACCCtrlAvail)  "<VOUTP_VMCACCCtrlAvail_flg>"
  [BOUTP_outputs] -> bus_selector25/1
  bus_selector26/1 -> VMCAEBCtrlAvail/1(VMCAEBCtrlAvail)  "<VOUTP_VMCAEBCtrlAvail_flg>"
  [BOUTP_outputs] -> bus_selector26/1
  bus_selector27/1 -> VMCCCCtrlAvail/1(VMCCCCtrlAvail)  "<VOUTP_VMCCCCtrlAvail_flg>"
  [BOUTP_outputs] -> bus_selector27/1
  bus_selector28/1 -> VMCMSACtrlAvail/1(VMCMSACtrlAvail)  "<VOUTP_VMCMSACtrlAvail_flg>"
  [BOUTP_outputs] -> bus_selector28/1
  bus_selector29/1 -> VMCVCUACCCtrlAvail/1(VMCVCUACCCtrlAvail)  "<VOUTP_ACCCtrlAvail_flg>"
  [BOUTP_outputs] -> bus_selector29/1
  bus_selector30/1 -> VMCVCUAPSCtrlAvailflg/1(VMCVCUAPSCtrlAvailflg)  "<VOUTP_APSCtrlAvail_flg>"
  [BOUTP_outputs] -> bus_selector30/1
  bus_selector31/1 -> VMCVCUAccPedalOverride/1(VMCVCUAccPedalOverride)  "<VOUTP_ACCPedalOvrd_flg>"
  [BOUTP_outputs] -> bus_selector31/1
  bus_selector32/1 -> VMCVCUCCCrlSta/1(VMCVCUCCCrlSta)  "<VOUTP_CCCtrlSta_enum>"
  [BOUTP_outputs] -> bus_selector32/1
  bus_selector33/1 -> VMCVCUMSACrlSta/1(VMCVCUMSACrlSta)  "<VOUTP_MSACtrlSta_enum>"
  [BOUTP_outputs] -> bus_selector33/1
  Ground/1 -> VehicleSpeedkph/1(VehicleSpeedkph)
  Ground1/1 -> VehicleSpeedmph/1(VehicleSpeedmph)

== system halout/HAL_OUT/CAN6/GW6_CE100_0_0x1C6 ==
  BSCP_outputs : Inport  OutDataTypeStr=Bus: BSCP_outputs
  BOUTP_outputs : Inport  Port=2  OutDataTypeStr=Bus: BOUTP_outputs
  FDCBCMDimSw : Subsystem
  FDCBCMFWipSwSta : Subsystem
  FDCBCMPassSWSta : Subsystem
  FDCBCMTurnSwSta : Subsystem
  FDCVMCSpdCtrlModeSta : Subsystem
  FDCVMCSpdCtrlSta : Subsystem
  bus_creator : BusCreator  Inputs=6  OutDataTypeStr=Bus: DT_CAN6_SG_GW6_CE100_0  NonVirtualBus=on
  bus_selector : BusSelector  OutputSignals=VOUTP_DimSwSta_flg
  bus_selector1 : BusSelector  OutputSignals=VOUTP_FWipSwSta_enum
  bus_selector2 : BusSelector  OutputSignals=VOUTP_PassSWSta_flg
  bus_selector3 : BusSelector  OutputSignals=VOUTP_TurnSwSta_enum
  bus_selector4 : BusSelector  OutputSignals=VOUTP_SpdCtrlMode_enum
  bus_selector5 : BusSelector  OutputSignals=VOUTP_SpdCtrlSta_flg
  GW6_CE100_0 : Outport
  wires:
  BSCP_outputs/1 -> [BSCP_outputs]
  BOUTP_outputs/1 -> [BOUTP_outputs]
  [CAN6_FDC_BCM_DimSw] -> bus_creator/1  "CAN6_FDC_BCM_DimSw"
  [CAN6_FDC_BCM_FWipSw_Sta] -> bus_creator/2  "CAN6_FDC_BCM_FWipSw_Sta"
  [CAN6_FDC_BCM_PassSW_Sta] -> bus_creator/3  "CAN6_FDC_BCM_PassSW_Sta"
  [CAN6_FDC_BCM_TurnSw_Sta] -> bus_creator/4  "CAN6_FDC_BCM_TurnSw_Sta"
  [CAN6_FDC_VMC_SpdCtrlMode_Sta] -> bus_creator/5  "CAN6_FDC_VMC_SpdCtrlMode_Sta"
  [CAN6_FDC_VMC_SpdCtrl_Sta] -> bus_creator/6  "CAN6_FDC_VMC_SpdCtrl_Sta"
  bus_creator/1 -> GW6_CE100_0/1
  FDCBCMDimSw/1(CAN6_FDC_BCM_DimSw) -> [CAN6_FDC_BCM_DimSw]
  FDCBCMFWipSwSta/1(CAN6_FDC_BCM_FWipSw_Sta) -> [CAN6_FDC_BCM_FWipSw_Sta]
  FDCBCMPassSWSta/1(CAN6_FDC_BCM_PassSW_Sta) -> [CAN6_FDC_BCM_PassSW_Sta]
  FDCBCMTurnSwSta/1(CAN6_FDC_BCM_TurnSw_Sta) -> [CAN6_FDC_BCM_TurnSw_Sta]
  FDCVMCSpdCtrlModeSta/1(CAN6_FDC_VMC_SpdCtrlMode_Sta) -> [CAN6_FDC_VMC_SpdCtrlMode_Sta]
  FDCVMCSpdCtrlSta/1(CAN6_FDC_VMC_SpdCtrl_Sta) -> [CAN6_FDC_VMC_SpdCtrl_Sta]
  bus_selector/1 -> FDCBCMDimSw/1(FDCBCMDimSw)  "<VOUTP_DimSwSta_flg>"
  [BOUTP_outputs] -> bus_selector/1
  bus_selector1/1 -> FDCBCMFWipSwSta/1(FDCBCMFWipSwSta)  "<VOUTP_FWipSwSta_enum>"
  [BOUTP_outputs] -> bus_selector1/1
  bus_selector2/1 -> FDCBCMPassSWSta/1(FDCBCMPassSWSta)  "<VOUTP_PassSWSta_flg>"
  [BOUTP_outputs] -> bus_selector2/1
  bus_selector3/1 -> FDCBCMTurnSwSta/1(FDCBCMTurnSwSta)  "<VOUTP_TurnSwSta_enum>"
  [BOUTP_outputs] -> bus_selector3/1
  bus_selector4/1 -> FDCVMCSpdCtrlModeSta/1(FDCVMCSpdCtrlModeSta)  "<VOUTP_SpdCtrlMode_enum>"
  [BOUTP_outputs] -> bus_selector4/1
  bus_selector5/1 -> FDCVMCSpdCtrlSta/1(FDCVMCSpdCtrlSta)  "<VOUTP_SpdCtrlSta_flg>"
  [BOUTP_outputs] -> bus_selector5/1

== system halout/HAL_OUT/CAN1/FD1_APS2_0x210/APSDFLL ==
  APSDFLL : Inport
  Data Type Conversion : DataTypeConversion  OutDataTypeStr=uint16  RndMeth=Round
  CAN1_APS_D_FLL : Outport
  wires:
  Data Type Conversion/1 -> CAN1_APS_D_FLL/1
  APSDFLL/1 -> Data Type Conversion/1

== system halout/HAL_OUT/CAN1/FD1_APS2_0x210/APSDFLR ==
  APSDFLR : Inport
  Data Type Conversion : DataTypeConversion  OutDataTypeStr=uint16  RndMeth=Round
  CAN1_APS_D_FLR : Outport
  wires:
  Data Type Conversion/1 -> CAN1_APS_D_FLR/1
  APSDFLR/1 -> Data Type Conversion/1

== system halout/HAL_OUT/CAN1/FD1_APS2_0x210/APSDRLL ==
  APSDRLL : Inport
  Data Type Conversion : DataTypeConversion  OutDataTypeStr=uint16  RndMeth=Round
  CAN1_APS_D_RLL : Outport
  wires:
  Data Type Conversion/1 -> CAN1_APS_D_RLL/1
  APSDRLL/1 -> Data Type Conversion/1

== system halout/HAL_OUT/CAN1/FD1_APS2_0x210/APSDRLR ==
  APSDRLR : Inport
  Data Type Conversion : DataTypeConversion  OutDataTypeStr=uint16  RndMeth=Round
  CAN1_APS_D_RLR : Outport
  wires:
  Data Type Conversion/1 -> CAN1_APS_D_RLR/1
  APSDRLR/1 -> Data Type Conversion/1

== system halout/HAL_OUT/CAN1/FD1_APS2_0x210/APSExitCondition ==
  APSExitCondition : Inport
  Data Type Conversion : DataTypeConversion  OutDataTypeStr=uint8  RndMeth=Round
  CAN1_APS_ExitCondition : Outport
  wires:
  Data Type Conversion/1 -> CAN1_APS_ExitCondition/1
  APSExitCondition/1 -> Data Type Conversion/1

== system halout/HAL_OUT/CAN1/FD1_APS2_0x210/APSHWVer ==
  APSHWVer : Inport
  Data Type Conversion : DataTypeConversion  OutDataTypeStr=uint8  RndMeth=Round
  CAN1_APS_HW_Ver : Outport
  wires:
  Data Type Conversion/1 -> CAN1_APS_HW_Ver/1
  APSHWVer/1 -> Data Type Conversion/1

== system halout/HAL_OUT/CAN1/FD1_APS2_0x210/APSProgressPCT ==
  APSProgressPCT : Inport
  Data Type Conversion : DataTypeConversion  OutDataTypeStr=uint8  RndMeth=Round
  CAN1_APS_Progress_PCT : Outport
  wires:
  Data Type Conversion/1 -> CAN1_APS_Progress_PCT/1
  APSProgressPCT/1 -> Data Type Conversion/1

== system halout/HAL_OUT/CAN1/FD1_APS2_0x210/APSRQDisplay ==
  APSRQDisplay : Inport
  Data Type Conversion : DataTypeConversion  OutDataTypeStr=uint8  RndMeth=Round
  CAN1_APS_RQ_Display : Outport
  wires:
  Data Type Conversion/1 -> CAN1_APS_RQ_Display/1
  APSRQDisplay/1 -> Data Type Conversion/1

== system halout/HAL_OUT/CAN1/FD1_APS2_0x210/APSSWVer ==
  APSSWVer : Inport
  Data Type Conversion : DataTypeConversion  OutDataTypeStr=uint8  RndMeth=Round
  CAN1_APS_SW_Ver : Outport
  wires:
  Data Type Conversion/1 -> CAN1_APS_SW_Ver/1
  APSSWVer/1 -> Data Type Conversion/1

== system halout/HAL_OUT/CAN1/FD1_APS2_0x210/PASAFCL ==
  PASAFCL : Inport
  Data Type Conversion : DataTypeConversion  OutDataTypeStr=uint8  RndMeth=Round
  CAN1_PAS_A_FCL : Outport
  wires:
  Data Type Conversion/1 -> CAN1_PAS_A_FCL/1
  PASAFCL/1 -> Data Type Conversion/1

== system halout/HAL_OUT/CAN1/FD1_APS2_0x210/PASAFCR ==
  PASAFCR : Inport
  Data Type Conversion : DataTypeConversion  OutDataTypeStr=uint8  RndMeth=Round
  CAN1_PAS_A_FCR : Outport
  wires:
  Data Type Conversion/1 -> CAN1_PAS_A_FCR/1
  PASAFCR/1 -> Data Type Conversion/1

== system halout/HAL_OUT/CAN1/FD1_APS2_0x210/PASAFML ==
  PASAFML : Inport
  Data Type Conversion : DataTypeConversion  OutDataTypeStr=uint8  RndMeth=Round
  CAN1_PAS_A_FML : Outport
  wires:
  Data Type Conversion/1 -> CAN1_PAS_A_FML/1
  PASAFML/1 -> Data Type Conversion/1

== system halout/HAL_OUT/CAN1/FD1_APS2_0x210/PASAFMR ==
  PASAFMR : Inport
  Data Type Conversion : DataTypeConversion  OutDataTypeStr=uint8  RndMeth=Round
  CAN1_PAS_A_FMR : Outport
  wires:
  Data Type Conversion/1 -> CAN1_PAS_A_FMR/1
  PASAFMR/1 -> Data Type Conversion/1

== system halout/HAL_OUT/CAN1/FD1_APS2_0x210/PASARCL ==
  PASARCL : Inport
  Data Type Conversion : DataTypeConversion  OutDataTypeStr=uint8  RndMeth=Round
  CAN1_PAS_A_RCL : Outport
  wires:
  Data Type Conversion/1 -> CAN1_PAS_A_RCL/1
  PASARCL/1 -> Data Type Conversion/1

== system halout/HAL_OUT/CAN1/FD1_APS2_0x210/PASARCR ==
  PASARCR : Inport
  Data Type Conversion : DataTypeConversion  OutDataTypeStr=uint8  RndMeth=Round
  CAN1_PAS_A_RCR : Outport
  wires:
  Data Type Conversion/1 -> CAN1_PAS_A_RCR/1
  PASARCR/1 -> Data Type Conversion/1

== system halout/HAL_OUT/CAN1/FD1_APS2_0x210/PASARML ==
  PASARML : Inport
  Data Type Conversion : DataTypeConversion  OutDataTypeStr=uint8  RndMeth=Round
  CAN1_PAS_A_RML : Outport
  wires:
  Data Type Conversion/1 -> CAN1_PAS_A_RML/1
  PASARML/1 -> Data Type Conversion/1

== system halout/HAL_OUT/CAN1/FD1_APS2_0x210/PASARMR ==
  PASARMR : Inport
  Data Type Conversion : DataTypeConversion  OutDataTypeStr=uint8  RndMeth=Round
  CAN1_PAS_A_RMR : Outport
  wires:
  Data Type Conversion/1 -> CAN1_PAS_A_RMR/1
  PASARMR/1 -> Data Type Conversion/1

== system halout/HAL_OUT/CAN1/FD1_APS2_0x210/PASChime ==
  PASChime : Inport
  Data Type Conversion : DataTypeConversion  OutDataTypeStr=uint8  RndMeth=Round
  CAN1_PAS_Chime : Outport
  wires:
  Data Type Conversion/1 -> CAN1_PAS_Chime/1
  PASChime/1 -> Data Type Conversion/1

== system halout/HAL_OUT/CAN1/FD1_APS2_0x210/PASDFCL ==
  PASDFCL : Inport
  Data Type Conversion : DataTypeConversion  OutDataTypeStr=uint8  RndMeth=Round
  CAN1_PAS_D_FCL : Outport
  wires:
  Data Type Conversion/1 -> CAN1_PAS_D_FCL/1
  PASDFCL/1 -> Data Type Conversion/1

== system halout/HAL_OUT/CAN1/FD1_APS2_0x210/PASDFCR ==
  PASDFCR : Inport
  Data Type Conversion : DataTypeConversion  OutDataTypeStr=uint8  RndMeth=Round
  CAN1_PAS_D_FCR : Outport
  wires:
  Data Type Conversion/1 -> CAN1_PAS_D_FCR/1
  PASDFCR/1 -> Data Type Conversion/1

== system halout/HAL_OUT/CAN1/FD1_APS2_0x210/PASDFML ==
  PASDFML : Inport
  Data Type Conversion : DataTypeConversion  OutDataTypeStr=uint8  RndMeth=Round
  CAN1_PAS_D_FML : Outport
  wires:
  Data Type Conversion/1 -> CAN1_PAS_D_FML/1
  PASDFML/1 -> Data Type Conversion/1

== system halout/HAL_OUT/CAN1/FD1_APS2_0x210/PASDFMR ==
  PASDFMR : Inport
  Data Type Conversion : DataTypeConversion  OutDataTypeStr=uint8  RndMeth=Round
  CAN1_PAS_D_FMR : Outport
  wires:
  Data Type Conversion/1 -> CAN1_PAS_D_FMR/1
  PASDFMR/1 -> Data Type Conversion/1

== system halout/HAL_OUT/CAN1/FD1_APS2_0x210/PASDRCL ==
  PASDRCL : Inport
  Data Type Conversion : DataTypeConversion  OutDataTypeStr=uint8  RndMeth=Round
  CAN1_PAS_D_RCL : Outport
  wires:
  Data Type Conversion/1 -> CAN1_PAS_D_RCL/1
  PASDRCL/1 -> Data Type Conversion/1

== system halout/HAL_OUT/CAN1/FD1_APS2_0x210/PASDRCR ==
  PASDRCR : Inport
  Data Type Conversion : DataTypeConversion  OutDataTypeStr=uint8  RndMeth=Round
  CAN1_PAS_D_RCR : Outport
  wires:
  Data Type Conversion/1 -> CAN1_PAS_D_RCR/1
  PASDRCR/1 -> Data Type Conversion/1
